simulink model "Model1_1_after"  (R2015a)
settings: Solver=ode45  StartTime=0.0  StopTime=10.0  RelTol=1e-3
settings Model: Creator=qiji  LastModifiedBy=qiji
settings DebuggingCC: UnderspecifiedInitializationDetection=Classic  MergeDetectMultiDrivingBlocksExec=none  SolverPrmCheckMsg=warning

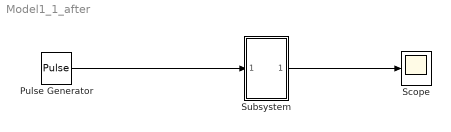
== system Model1_1_after ==
  Pulse Generator : DiscretePulseGenerator  Period=5
  Scope : Scope
  Subsystem : Subsystem
  wires:
  Pulse Generator/1 -> Subsystem/1(In1)
  Subsystem/1(Out) -> Scope/1

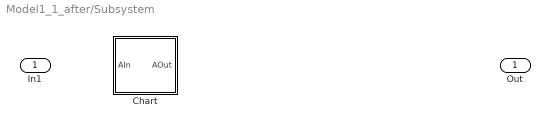
== system Model1_1_after/Subsystem ==
  In1 : Inport
  Chart : Stateflow chart  TreatAsAtomicUnit=on
  Out : Outport

== stateflow chart Model1_1_after/Subsystem/Chart ==
  state A
    en:
    AOut = 0;
  state B
    en:
    AOut = 1;
  A -> B : [AIn == 1]
  (default) -> A
  B -> A : [AIn==1]
  data: AIn input double; AOut output double
